simulink model "observadorminimo"  (R2021b)
settings: Solver=VariableStepAuto  StartTime=0.0  StopTime=10.0  RelTol=1e-3
values from neighbouring files (symbols this model uses):
  A = sys.A    [RealEstadoObserServoTipo0.m]
  B = sys.B    [RealEstadoObserServoTipo0.m]
  C = sys.C    [RealEstadoObserServoTipo0.m]    (also in control 2 tf.mat = 0.0033)
  K = Khat(1:m-1)    [RealEstadoObserServoTipo0.m]
  Ke = acker(A',C',[-30 -30 -30])'    [RealEstadoObserServoTipo0.m]
settings Model: Creator=57321  LastModifiedBy=57321

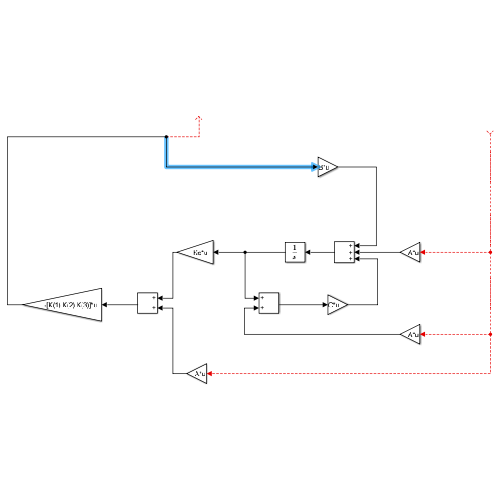
[thumbnail: Simulink's stored preview of the top-level diagram]
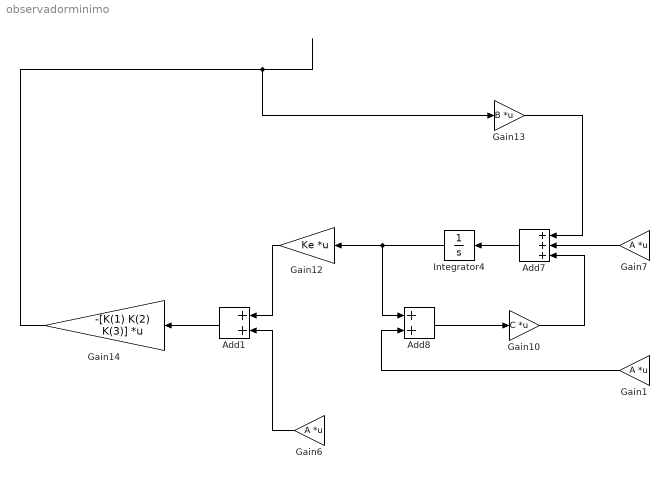
== system observadorminimo ==
  Add1 : Sum
  Add7 : Sum  Inputs=+++
  Add8 : Sum
  Gain1 : Gain  Gain=A  Multiplication=Matrix(K*u)
  Gain10 : Gain  Gain=C  Multiplication=Matrix(K*u)
  Gain12 : Gain  Gain=Ke  Multiplication=Matrix(K*u)
  Gain13 : Gain  Gain=B  Multiplication=Matrix(K*u)
  Gain14 : Gain  Gain=-[K(1) K(2) K(3)]  Multiplication=Matrix(K*u)
  Gain6 : Gain  Gain=A  Multiplication=Matrix(K*u)
  Gain7 : Gain  Gain=A  Multiplication=Matrix(K*u)
  Integrator4 : Integrator  InitialCondition=[0;0;0]
  wires:
  Gain13/1 -> Add7/1
  Gain7/1 -> Add7/2
  ? -> Gain7/1, Gain1/1, Gain6/1
  Gain10/1 -> Add7/3
  Add7/1 -> Integrator4/1
  Integrator4/1 -> Add8/1, Gain12/1
  Add8/1 -> Gain10/1
  Gain6/1 -> Add1/2
  Gain12/1 -> Add1/1
  Add1/1 -> Gain14/1
  Gain1/1 -> Add8/2
  Gain14/1 -> Gain13/1
